simulink model "RECDCDCclosedloopINV"  (R2015a)
settings: Solver=ode23tb  StartTime=0.0  StopTime=1  RelTol=1e-3
libraries: powerlib x38, simulink x2, simulink_extras x1
settings Model: Creator=vishn  LastModifiedBy=Ratish Kumar S

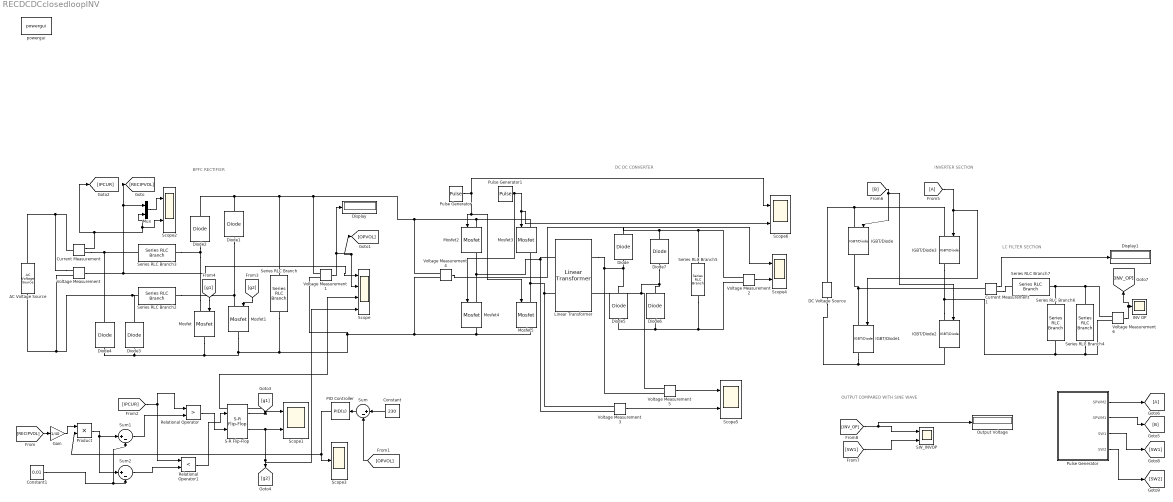
== system RECDCDCclosedloopINV ==
  note: DC DC CONVERTER
  note: BPFC RECTIFIER
  note: OUTPUT COMPARED WITH
      | SINE WAVE
  note: INVERTER SECTION
  note: LC FILTER SECTION
  AC Voltage Source : powerlib/Electrical Sources/AC Voltage Source  Amplitude=230  Phase=0  Frequency=50  SampleTime=0  Measurements=None
  Constant : Constant  Value=230
  Constant1 : Constant  Value=0.01
  Current Measurement : powerlib/Measurements/Current Measurement  PhasorSimulation=off  OutputType=Complex  PSBequivalent=0
  Current Measurement1 : powerlib/Measurements/Current Measurement  PhasorSimulation=off  OutputType=Complex  PSBequivalent=0
  DC Voltage Source : powerlib/Electrical Sources/DC Voltage Source  Amplitude=100  Measurements=None
  Diode{,1..7} (8 alike) : powerlib/Power Electronics/Diode  Ron=0.001  Lon=0  Vf=0.8  IC=0  UseSnubber=off  Rs=500  Cs=250e-9  Measurements=off
  Display : Display
  Display1 : Display
  Gain : Gain  Gain=1/40
  IGBT/Diode{,1..3} (4 alike) : powerlib/Power Electronics/IGBT//Diode  Ron=1e-3  Rs=1e5  Cs=inf  Measurements=on
  INV OP : Scope
      settings: TimeRange=1  YMin=-300  YMax=300  SaveName=ScopeData7
  Linear Transformer : powerlib/Elements/Linear Transformer  UNITS=SI  NominalPower=[5e3 50000 ]  winding1=[230 0.0004 0]  winding2=[230 0.0004 0]  ThreeWindings=off  winding3=[3.15e+05 24806 7.8961]  RmLm=[1000 21.518e-6]  Measurements=None  DataType=on
  Mosfet : powerlib/Power Electronics/Mosfet  Ron=0.1  Lon=0  Rd=0.01  Vfd=0  IC=0  Rs=1e5  Cs=inf  Measurements=off
  Mosfet1 : powerlib/Power Electronics/Mosfet  Ron=0.1  Lon=0  Rd=0.01  Vfd=0  IC=0  Rs=1e5  Cs=inf  Measurements=off
  Mosfet{2..5} (4 alike) : powerlib/Power Electronics/Mosfet  Ron=2e-3  Lon=0  Rd=2e-3  Vfd=1  IC=0  Rs=1e5  Cs=inf  Measurements=on
  Mux : Mux  Inputs=2
  Output Voltage : Display
  PID Controller : simulink/Continuous/PID Controller  Controller=PID  TimeDomain=Continuous-time  SampleTime=-1  IntegratorMethod=Forward Euler  FilterMethod=Forward Euler  Form=Parallel  UseFilter=on  ControllerParametersSource=internal  P=-0.01  I=1  D=7.5  N=1  InitialConditionSource=internal  InitialConditionForIntegrator=0  InitialConditionForFilter=0  ExternalReset=none  ZeroCross=off  LimitOutput=off  UpperSaturationLimit=inf  LowerSaturationLimit=-inf  LinearizeAsGain=on  AntiWindupMode=none  Kb=1  TrackingMode=off  Kt=1  PParamMin=[]  PParamMax=[]  IParamMin=[]  IParamMax=[]  DParamMin=[]  DParamMax=[]  NParamMin=[]  NParamMax=[]  KbParamMin=[]  KbParamMax=[]  KtParamMin=[]  KtParamMax=[]  POutMin=[]  POutMax=[]  IOutMin=[]  IOutMax=[]  DOutMin=[]  DOutMax=[]  NOutMin=[]  NOutMax=[]  KbOutMin=[]  KbOutMax=[]  KtOutMin=[]  KtOutMax=[]  IntegratorOutMin=[]  IntegratorOutMax=[]  FilterOutMin=[]  FilterOutMax=[]  SumOutMin=[]  SumOutMax=[]  SumI1OutMin=[]  SumI1OutMax=[]  SumI2OutMin=[]  SumI2OutMax=[]  SumI3OutMin=[]  SumI3OutMax=[]  SumDOutMin=[]  SumDOutMax=[]  SaturationOutMin=[]  SaturationOutMax=[]  IntegratorContinuousStateAttributes=''  IntegratorStateMustResolveToSignalObject=off  IntegratorRTWStateStorageClass=Auto  FilterContinuousStateAttributes=''  FilterStateMustResolveToSignalObject=off  FilterRTWStateStorageClass=Auto  DifferentiatorICPrevScaledInput=0  DifferentiatorOutMin=[]  DifferentiatorOutMax=[]
  Product : Product
  Pulse Generator : DiscretePulseGenerator  PulseType=Time based  Period=.00002  PulseWidth=50  VectorParams1D=off
  Pulse Generator1 : DiscretePulseGenerator  PulseType=Time based  Period=.00002  PulseWidth=50  PhaseDelay=2.22e-10  VectorParams1D=off
  "Pulse Generator " : Subsystem
  Relational Operator : RelationalOperator  Operator=>  OutDataTypeStr=boolean
  Relational Operator1 : RelationalOperator  Operator=<  OutDataTypeStr=boolean
  S-R Flip-Flop : simulink_extras/Flip Flops/S-R Flip-Flop  initial_condition=0
  SW_INVOP : Scope  NumInputPorts=2
      settings: YMin=-250~-0.8  YMax=250~0.8  SaveName=ScopeData8
  Scope : Scope  NumInputPorts=4
      settings: YMin=-250~543.9~0~0  YMax=250~543.96~1~1
  Scope{1..2,4..6} (5 alike) : Scope  NumInputPorts=2
      Scope1 settings: TimeRange=0.7926773900484776  YMin=-0.125~-0.125  YMax=1.125~1.125
      Scope2 settings: TimeRange=0.7926773900484776  YMin=-4752.32749~-4750.58513  YMax=528.03639~512.35513  SaveName=ScopeData2
      Scope4 settings: TimeRange=0.1  YMin=25~40  YMax=225~200  SaveName=ScopeData4  Decimation=20
      Scope5 settings: YMin=105~105  YMax=145~147.5  SaveName=ScopeData5  Decimation=20
      Scope6 settings: YMin=-1~-1  YMax=6~6  SaveName=ScopeData6  Decimation=20
  Scope3 : Scope
      settings: YMin=175  YMax=475  SaveName=ScopeData3
  Series RLC Branch : powerlib/Elements/Series RLC Branch  LConnTagsString=__new0  RConnTagsString=__new0  BranchType=C  Resistance=1  Inductance=1e-3  SetiL0=off  InitialCurrent=0  Capacitance=1000e-6  Setx0=off  InitialVoltage=0  Measurements=None
  Series RLC Branch2 : powerlib/Elements/Series RLC Branch  LConnTagsString=__new0  RConnTagsString=__new0  BranchType=L  Resistance=1  Inductance=5e-3  SetiL0=off  InitialCurrent=0  Capacitance=1e-6  Setx0=off  InitialVoltage=0  Measurements=None
  Series RLC Branch3 : powerlib/Elements/Series RLC Branch  LConnTagsString=__new0  RConnTagsString=__new0  BranchType=L  Resistance=1  Inductance=5e-3  SetiL0=off  InitialCurrent=0  Capacitance=1e-6  Setx0=off  InitialVoltage=0  Measurements=None
  Series RLC Branch4 : powerlib/Elements/Series RLC Branch  LConnTagsString=__new0  RConnTagsString=__new0  BranchType=R  Resistance=50  Inductance=40e-3  SetiL0=off  InitialCurrent=0  Capacitance=500e-3  Setx0=off  InitialVoltage=0  Measurements=None
  Series RLC Branch5 : powerlib/Elements/Series RLC Branch  LConnTagsString=__new0  RConnTagsString=__new0  BranchType=C  Resistance=1  Inductance=1e-3  SetiL0=off  InitialCurrent=0  Capacitance=500e-6  Setx0=off  InitialVoltage=0  Measurements=Branch voltage
  Series RLC Branch6 : powerlib/Elements/Series RLC Branch  LConnTagsString=__new0  RConnTagsString=__new0  BranchType=C  Resistance=1  Inductance=40e-3  SetiL0=off  InitialCurrent=0  Capacitance=1.9e-4  Setx0=off  InitialVoltage=0  Measurements=None
  Series RLC Branch7 : powerlib/Elements/Series RLC Branch  LConnTagsString=__new0  RConnTagsString=__new0  BranchType=L  Resistance=1  Inductance=500e-4  SetiL0=off  InitialCurrent=0  Capacitance=500e-3  Setx0=off  InitialVoltage=0  Measurements=None
  Sum : Sum  Inputs=|+-
  Sum1 : Sum  Inputs=|+-
  Sum2 : Sum  Inputs=|+-
  Voltage Measurement{,1..6} (7 alike) : powerlib/Measurements/Voltage Measurement  PhasorSimulation=off  OutputType=Complex  PSBequivalent=0
  powergui : powerlib/powergui  Priority=1  SimulationMode=Discrete  SolverType=Tustin/Backward Euler (TBE)  SampleTime=1e-6  frequency=60  SPID=off  DisableSnubberDevices=off  DisableRonSwitches=off  DisableVfSwitches=off  SwTol=0  DisplayEquations=off  Interpol=off  methode=off  Ts=100  FunctionMessages=off  echomessages=off  HookPort=off  EnableUseOfTLC=off  x0status=blocks  frequencyindice=0  Pbase=100e6  ErrMax=1e-4  Iterations=50  UnitsV=kV  UnitsW=MW  buscounter=0  RestoreLinks=warning  ResistiveCurrentMeasurement=off  Frange=[0:2:500]  Ylog=off  Xlog=on  ShowGrid=off  save=off  variable=ZData  structure=0  ZoomFFT=off  StartTime=0.0  cycles=1  DisplayStyle=1  fundamental=60  FreqAxis=off  MaxFrequency=1000  frequencyindicesteady=1  RmsSteady=1  display=off
  wires:
  Voltage Measurement/1 -> Scope/1, [RECIPVOL], Mux/1
  Voltage Measurement1/1 -> Scope/2, [OPVOL], Display/1
  [OPVOL] -> Sum/2
  Constant/1 -> Sum/1
  Sum/1 -> PID Controller/1
  Current Measurement/1 -> Scope2/2, Mux/2, [IPCUR]
  [RECIPVOL] -> Gain/1
  [IPCUR] -> Relational Operator/1, Relational Operator1/1
  Constant1/1 -> Sum1/2, Sum2/2
  Sum2/1 -> Relational Operator1/2
  Sum1/1 -> Relational Operator/2
  Relational Operator/1 -> S-R Flip-Flop/2
  Relational Operator1/1 -> S-R Flip-Flop/1
  S-R Flip-Flop/1 -> Scope/3, Scope1/1, [g1]
  S-R Flip-Flop/2 -> [g2], Scope/4, Scope1/2
  [g1] -> Mosfet/1
  [g2] -> Mosfet1/1
  Product/1 -> Sum2/1, Sum1/1
  Gain/1 -> Product/1
  PID Controller/1 -> Scope3/1, Product/2
  Mux/1 -> Scope2/1
  Pulse Generator/1 -> Scope6/1, Mosfet2/1, Mosfet5/1
  Pulse Generator1/1 -> Scope6/2, Mosfet3/1, Mosfet4/1
  Voltage Measurement4/1 -> Scope4/1
  Voltage Measurement3/1 -> Scope5/2
  Voltage Measurement5/1 -> Scope5/1
  Voltage Measurement2/1 -> Scope4/2
  [A] -> IGBT/Diode1/1, IGBT/Diode3/1
  Voltage Measurement6/1 -> [INV_OP], INV OP/1
  [INV_OP] -> Output Voltage/1, SW_INVOP/1
  [SW1] -> SW_INVOP/2
  Current Measurement1/1 -> Display1/1
  "Pulse Generator "/1(SPWM2) -> [A]
  "Pulse Generator "/2(SPWM1) -> [B]
  [B] -> IGBT/Diode/1, IGBT/Diode2/1
  "Pulse Generator "/3(SW1) -> [SW1]
  "Pulse Generator "/4(SW2) -> [SW2]
  connections:
  Mosfet3/LConn1 -- Voltage Measurement4/LConn1 -- Diode2/RConn1 -- Diode1/RConn1 -- Series RLC Branch/LConn1 -- Voltage Measurement1/LConn1 -- Mosfet2/LConn1
  Voltage Measurement/LConn1 -- Current Measurement/LConn1 -- AC Voltage Source/RConn1
  Series RLC Branch2/RConn1 -- Mosfet1/LConn1 -- Diode1/LConn1
  Mosfet5/RConn1 -- Voltage Measurement4/LConn2 -- Series RLC Branch/RConn1 -- Diode3/LConn1 -- Diode4/LConn1 -- Mosfet/RConn1 -- Mosfet1/RConn1 -- Voltage Measurement1/LConn2 -- Mosfet4/RConn1
  Diode2/LConn1 -- Series RLC Branch3/RConn1 -- Mosfet/LConn1
  Diode4/RConn1 -- Current Measurement/RConn1 -- Series RLC Branch3/LConn1
  Voltage Measurement/LConn2 -- Diode3/RConn1 -- Series RLC Branch2/LConn1 -- AC Voltage Source/LConn1
  Mosfet3/RConn1 -- Mosfet5/LConn1 -- Linear Transformer/LConn2 -- Voltage Measurement3/LConn1
  Voltage Measurement5/LConn1 -- Diode6/RConn1 -- Diode7/LConn1 -- Linear Transformer/RConn2
  Diode/LConn1 -- Linear Transformer/RConn1 -- Voltage Measurement5/LConn2 -- Diode5/RConn1
  Mosfet2/RConn1 -- Mosfet4/LConn1 -- Voltage Measurement3/LConn2 -- Linear Transformer/LConn1
  IGBT/Diode1/RConn1 -- IGBT/Diode2/RConn1 -- DC Voltage Source/LConn1
  Series RLC Branch7/LConn1 -- Series RLC Branch6/LConn1 -- Series RLC Branch4/LConn1 -- Voltage Measurement6/LConn1
  IGBT/Diode/RConn1 -- IGBT/Diode1/LConn1 -- Current Measurement1/LConn1
  IGBT/Diode2/LConn1 -- IGBT/Diode3/RConn1 -- Voltage Measurement6/LConn2 -- Series RLC Branch4/RConn1 -- Series RLC Branch6/RConn1
  Current Measurement1/RConn1 -- Series RLC Branch7/RConn1
  IGBT/Diode/LConn1 -- IGBT/Diode3/LConn1 -- DC Voltage Source/RConn1
  Series RLC Branch5/LConn1 -- Voltage Measurement2/LConn1 -- Diode/RConn1 -- Diode7/RConn1
  Voltage Measurement2/LConn2 -- Series RLC Branch5/RConn1 -- Diode6/LConn1 -- Diode5/LConn1

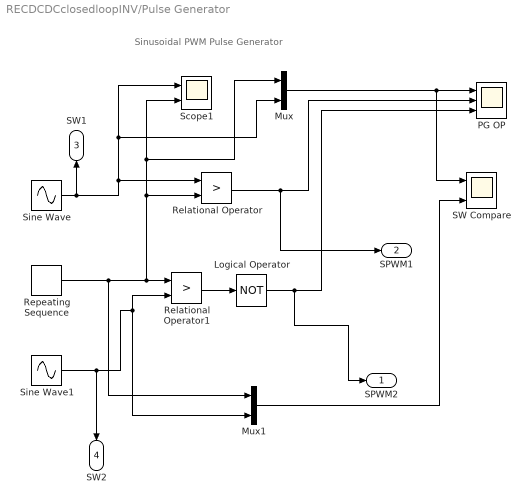
== system RECDCDCclosedloopINV/Pulse Generator  ==
  note: Sinusoidal PWM Pulse Generator
  Logical Operator : Logic  Operator=NOT  AllPortsSameDT=off  OutDataTypeStr=boolean
  Mux : Mux  Inputs=2
  Mux1 : Mux  Inputs=2
  PG OP : Scope  NumInputPorts=3
      settings: YMin=-10~-5~-5  YMax=10~5~5
  Relational Operator : RelationalOperator  Operator=>  OutDataTypeStr=boolean
  Relational Operator1 : RelationalOperator  Operator=>  OutDataTypeStr=boolean
  Repeating Sequence : simulink/Sources/Repeating Sequence  rep_seq_t=[0 0.5 1]*(1/1000)  rep_seq_y=[0 1 0]
  SW Compare : Scope  NumInputPorts=2
      settings: YMin=-10~-5  YMax=10~5  SaveName=ScopeData3
  Scope1 : Scope  NumInputPorts=2
      settings: YMin=-5~-5  YMax=5~5
  Sine Wave : Sin  Amplitude=0.8  Frequency=2*pi*50  SampleTime=0
  Sine Wave1 : Sin  Amplitude=0.8  Frequency=2*pi*50  Phase=pi  SampleTime=0
  SPWM2 : Outport
  SPWM1 : Outport  Port=2
  SW1 : Outport  Port=3
  SW2 : Outport  Port=4
  wires:
  Mux1/1 -> SW Compare/2
  Sine Wave/1 -> SW1/1, Relational Operator/1, Mux/2, Scope1/1
  Relational Operator/1 -> SPWM1/1, PG OP/2
  Mux/1 -> PG OP/1, SW Compare/1
  Sine Wave1/1 -> SW2/1, Mux1/2, Relational Operator1/2
  Repeating Sequence/1 -> Mux1/1, Relational Operator/2, Mux/1, Scope1/2, Relational Operator1/1
  Relational Operator1/1 -> Logical Operator/1
  Logical Operator/1 -> SPWM2/1, PG OP/3
